simulink model "Biosimp3"  (R2016b)
settings: Solver=ode2  StartTime=0.0  StopTime=300  FixedStep=0.1  RelTol=1e-3
values from neighbouring files (symbols this model uses):
  Cm = 20    [MotorNeuron.m]    (also in nullclines.m; nullclinesk.m)
  fai_Ca = 0.1    [MotorNeuron.m]
  fai_K = 0.067    [MotorNeuron.m]
  g_Ca = 40    [MotorNeuron.m]    (also in nullclines.m = 100; nullclinesk.m = 100)
  g_K = 0    [MotorNeuron.m]    (also in nullclines.m = 8; nullclinesk.m = 8)
  g_L = 2    [MotorNeuron.m]    (also in nullclines.m = 3; nullclinesk.m = 3)
  V1 = 0    [MotorNeuron.m]    (also in nullclines.m = -1; nullclinesk.m = -1)
  V2 = 15    [MotorNeuron.m]    (also in nullclines.m; nullclinesk.m)
  V3 = 10    [MotorNeuron.m]    (also in nullclines.m = -1; nullclinesk.m = -1)
  V4 = 10    [MotorNeuron.m]    (also in nullclines.m = 14.5; nullclinesk.m = 14.5)
  V_Ca = 30    [MotorNeuron.m]    (also in nullclines.m = 0; nullclinesk.m = 100)
  V_K = -70    [MotorNeuron.m]    (also in nullclines.m = -150; nullclinesk.m = 0)
  V_L = -50    [MotorNeuron.m]    (also in nullclines.m; nullclinesk.m)
libraries: simulink x1
settings Model: Creator=User  LastModifiedBy=User

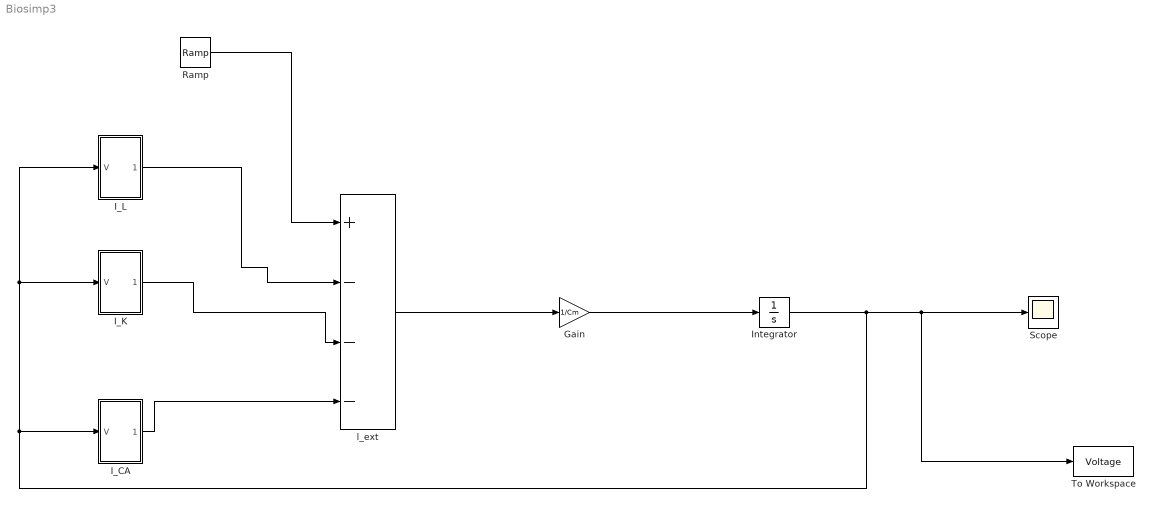
== system Biosimp3 ==
  Gain : Gain  Gain=1/Cm
  I_CA : Subsystem
  I_K : Subsystem
  I_L : Subsystem
  Integrator : Integrator  InitialCondition=-50
  Ramp : simulink/Sources/Ramp  slope=1  start=0  X0=15
  Scope : Scope
  To Workspace : ToWorkspace  VariableName=Voltage  SaveFormat=Timeseries  SampleTime=-1
  l_ext : Sum  Inputs=+---
  wires:
  I_L/1(Out1) -> l_ext/2
  I_K/1(Out1) -> l_ext/3
  I_CA/1(Out1) -> l_ext/4
  l_ext/1 -> Gain/1
  Gain/1 -> Integrator/1
  Integrator/1 -> To Workspace/1, Scope/1, I_CA/1(V), I_K/1(V), I_L/1(V)
  Ramp/1 -> l_ext/1

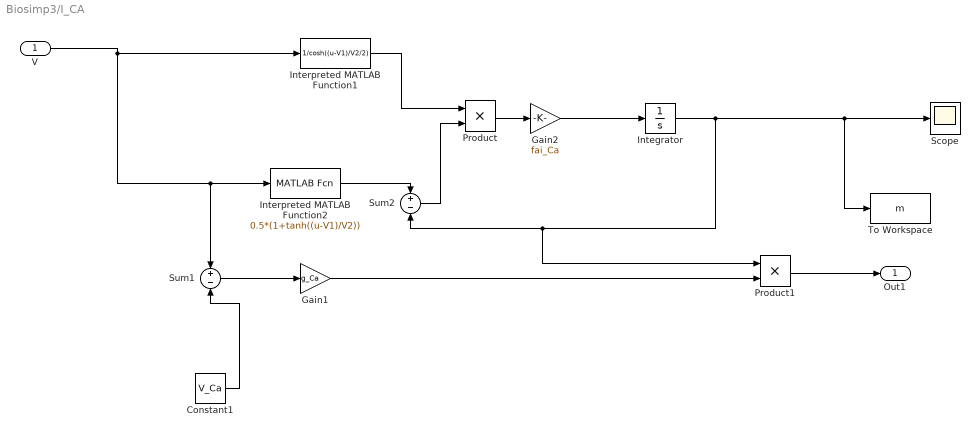
== system Biosimp3/I_CA ==
  V : Inport  OutMin=-10
  Constant1 : Constant  Value=V_Ca
  Gain1 : Gain  Gain=g_Ca
  Gain2 : Gain  Gain=fai_Ca
  Integrator : Integrator
  Interpreted MATLAB Function1 : MATLABFcn  MATLABFcn=1/cosh((u-V1)/V2/2)
  Interpreted MATLAB Function2 : MATLABFcn  MATLABFcn=0.5*(1+tanh((u-V1)/V2))
  Product : Product
  Product1 : Product
  Scope : Scope
  Sum1 : Sum  Inputs=+-
  Sum2 : Sum  Inputs=+-
  To Workspace : ToWorkspace  VariableName=m  SaveFormat=Timeseries  SampleTime=-1
  Out1 : Outport
  wires:
  Gain2/1 -> Integrator/1
  Gain1/1 -> Product1/2
  Constant1/1 -> Sum1/2
  Interpreted MATLAB Function1/1 -> Product/1
  Integrator/1 -> Product1/1, Sum2/2, To Workspace/1, Scope/1
  V/1 -> Interpreted MATLAB Function1/1, Sum1/1, Interpreted MATLAB Function2/1
  Sum1/1 -> Gain1/1
  Sum2/1 -> Product/2
  Interpreted MATLAB Function2/1 -> Sum2/1
  Product1/1 -> Out1/1
  Product/1 -> Gain2/1

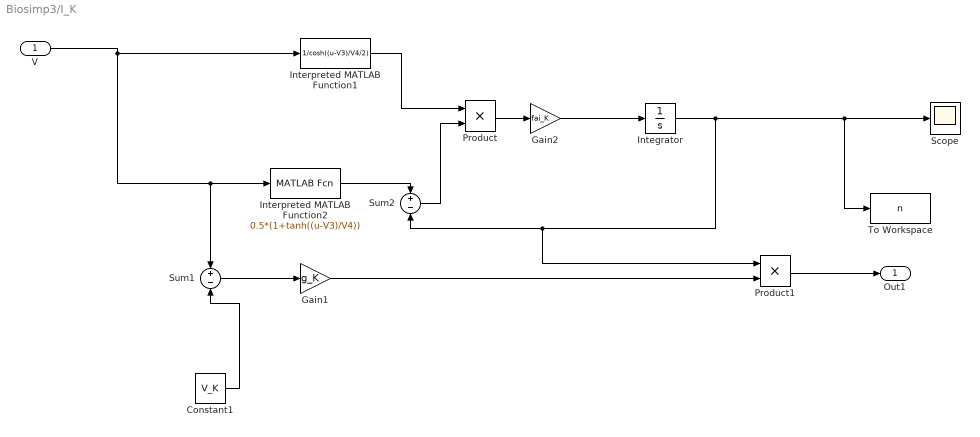
== system Biosimp3/I_K ==
  V : Inport  OutMin=-10
  Constant1 : Constant  Value=V_K
  Gain1 : Gain  Gain=g_K
  Gain2 : Gain  Gain=fai_K
  Integrator : Integrator
  Interpreted MATLAB Function1 : MATLABFcn  MATLABFcn=1/cosh((u-V3)/V4/2)
  Interpreted MATLAB Function2 : MATLABFcn  MATLABFcn=0.5*(1+tanh((u-V3)/V4))
  Product : Product
  Product1 : Product
  Scope : Scope
  Sum1 : Sum  Inputs=+-
  Sum2 : Sum  Inputs=+-
  To Workspace : ToWorkspace  VariableName=n  SaveFormat=Timeseries  SampleTime=-1
  Out1 : Outport
  wires:
  Gain2/1 -> Integrator/1
  Gain1/1 -> Product1/2
  Constant1/1 -> Sum1/2
  Interpreted MATLAB Function1/1 -> Product/1
  Integrator/1 -> Product1/1, Sum2/2, To Workspace/1, Scope/1
  V/1 -> Interpreted MATLAB Function1/1, Sum1/1, Interpreted MATLAB Function2/1
  Sum1/1 -> Gain1/1
  Sum2/1 -> Product/2
  Interpreted MATLAB Function2/1 -> Sum2/1
  Product1/1 -> Out1/1
  Product/1 -> Gain2/1

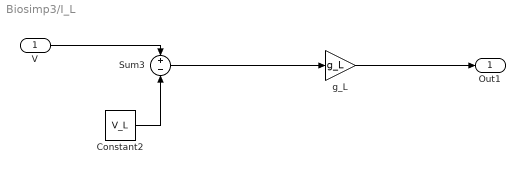
== system Biosimp3/I_L ==
  V : Inport  OutMin=-10
  Constant2 : Constant  Value=V_L
  Sum3 : Sum  Inputs=+-
  g_L : Gain  Gain=g_L
  Out1 : Outport
  wires:
  g_L/1 -> Out1/1
  Sum3/1 -> g_L/1
  Constant2/1 -> Sum3/2
  V/1 -> Sum3/1
